simulink model "Test_Schnittstelle"  (R2018a)
settings: Solver=FixedStepAuto  StartTime=0.0  StopTime=inf  FixedStep=0.0000001  RelTol=1e-3
model workspace (MAT data in the model file):
  MCOS : class17 (value not decoded)
  MCOS : class17 (value not decoded)
  MCOS : class17 (value not decoded)
  MCOS : class17 (value not decoded)
  MCOS : class17 (value not decoded)
  MCOS : class17 (value not decoded)
  MCOS : class17 (value not decoded)
  MCOS : class17 (value not decoded)
  MCOS : class17 (value not decoded)
  MCOS : class17 (value not decoded)
  MCOS : class17 (value not decoded)
  MCOS : class17 (value not decoded)
  MCOS : class17 (value not decoded)
  MCOS : class17 (value not decoded)
  MCOS : class17 (value not decoded)
(part 2 of 2)

== matlab function Test_Schnittstelle/Schnittstelle_0/Recv_2 ==
  data: status input double size=1; clock input double size=1; lenS_1 input; lenS_2 input; lenR input; Rx_2_signal input boolean size=1; Rx_2_data input double size=[1 100]; recv_signal_2 output boolean; recv_package_2 output double size=[1 98]; Send_Buffer_1 data_store_memory; Send_Buffer_2 data_store_memory; T_send_2 data_store_memory; T_recv_2 data_store_memory; De_2 data_store_memory; De_sum_1 data_store_memory; Address data_store_memory; Recv_Buffer data_store_memory; Address_2 data_store_memory; Address_1 data_store_memory; De_sum_2 data_store_memory; Handshake_2 data_store_memory
% Name: Rx_2

% Funktionalitäten:
% Im Init-Prozess
%   1. Handshake durch zu führen
%       103...Handshake ask --> 104 in Send_Buffer_1 additieren
%       104...Handshake answer --> Handshake success
%   2. Delay-Zeit berechnen
%       105...Delay begin --> 106 in Send_Buffer_1 additieren
%       106...Delay end --> Delay_Zeit berechnen
%   3. Sum-Delay-Zeit berechnen
%       107, Receiver = meine Addresse --> Sum_Delay_Zeit berechnen
%       107, Receiver ~= meine Addresse --> Daten in Send_Buffer_2 additieren
% Im normalen Prozess
%   4. Receiver = meine Addresse --> in Recv_Buffer additieren
%   5. Receiver = 255 --> Broadcast --> in Recv_Buffer && Send_Buffer_2 additieren
%   6. Receiver ~= meine Addresse --> in Send_Buffer_2 additieren

function [recv_signal_2, recv_package_2] = Rx_2(status, clock,lenS_1, lenS_2, lenR, Rx_2_signal, Rx_2_data)

global Send_Buffer_2
global Send_Buffer_1
global T_send_2
global T_recv_2
global De_2
global De_sum_2
global Address
global Address_2
%global Address_1
global Recv_Buffer
global Handshake_2

recv_signal_2 = false;
recv_package_2 = zeros(1,98);       % one datablock = [1x7]

lenr = 1;                           % path to write data into recv_package_2

if Rx_2_signal
    a = find(Rx_2_data==102,1);
    len = a(1);
    if ~isempty(len)
        mod_ = mod(len-2,7);
        len_ = ceil((len - 2) / 7);                                 % Round toward positive infinity
    end
    
	if ((mod_ == 0) && (len_ >= 1))                             % package contains at least one datablock
        switch status
            case 1                                              % Handshake
                for i=1:len_
                    switch Rx_2_data(7*i-3)                          % Da.cmd
                        case 103                                % Handshake ask --> send answer
                            check = check_X(104, Address, Send_Buffer_1);
                            if ((Rx_2_data(7*i-5) ~= 0) && (Rx_2_data(7*i-4) == 0) && ~Handshake_2 && ~check)
                                Address_2 = Rx_2_data(7*i-5);
                                Send_Buffer_1(lenS_1:lenS_1+7) = [Address, Address_2, 104, zeros(1,4), 102];
                            end
                        case 104                                % Handshake answer --> Handshake success --> no more send
                            if ((Rx_2_data(7*i-5) ~= 0) && (Rx_2_data(7*i-4) == Address) && ~Handshake_2)
                                Address_2 = Rx_2_data(7*i-5);        % Address of the Host in the Direction_2
                                recv_package_2(lenr:lenr+6) = Rx_2_data(7*i-5:7*i+1);    % [_,_,104,_,_,_,_] = [1x7]
                                lenr = lenr + 7;
                                recv_signal_2 = true;
                            end
                    end
                end

            case 2                                              % Delay_Time_Caculation
                for j=1:len_
                    switch Rx_2_data(7*j-3)                          % Da.cmd
                        case 103                                % Handshake ask --> send answer
                            check = check_X(104, Address, Send_Buffer_1);
                            if ((Rx_2_data(7*j-5) ~= 0) && (Rx_2_data(7*j-4) == 0) && ~Handshake_2 && ~check)
                                Address_2 = Rx_2_data(7*j-5);
                                Send_Buffer_1(lenS_1:lenS_1+7) = [Address, Address_2, 104, zeros(1,4), 102];
                            end
                        case 105                                % Delay ask --> send answer
                            check = check_X(106, Address, Send_Buffer_1);
                            if (isequal(Rx_2_data(7*j-5:7*j-4),[Address_2, Address]) && Handshake_2 && ~check) % check Sender & Receiver
                                Send_Buffer_1(lenS_1:lenS_1+7) = [Address, 0, 106, zeros(1,4), 102];
                            end
                        case 106                                % Delay answer --> caculate the time --> no more send
                            if ((isequal(Rx_2_data(7*j-5:7*j-3),[Address_2, Address, 106])) && (De_2 <= 0))
                                T_recv_2 = clock;
                                De_2 = T_recv_2 - T_send_2;
                                T_send_2 = 0;
                                T_recv_2 = 0;
                            end
                    end
                end

            case 3                                              % Sum_Delay_Caculation
                for h=1:len_
                    switch Rx_2_data(7*h-3)
                        case 103                                % Handshake ask --> send answer
                            check = check_X(104, Address, Send_Buffer_1);
                            if ((Rx_2_data(7*h-5) ~= 0) && (Rx_2_data(7*h-4) == 0) && ~Handshake_2 && ~check)
                                Address_2 = Rx_2_data(7*h-5);
                                Send_Buffer_1(lenS_1:lenS_1+7) = [Address, Address_2, 104, zeros(1,4), 102];
                            end
                        case 105                                % Delay ask --> send answer
                            check = check_X(106, Address, Send_Buffer_1);
                            if (isequal(Rx_2_data(7*h-5:7*h-4),[Address_2, Address]) && Handshake_2 && ~check) % check Sender & Receiver
                                Send_Buffer_1(lenS_1:lenS_1+7) = [Address, 0, 106, zeros(1,4), 102];
                            end   
                        case 107
                            if (isequal(Rx_2_data(7*h-5:7*h-4),[Address, Address]) && (De_sum_2 <= De_2))                   % Sum_Delay --> caculate the time --> no more send
                                T_recv_2 = clock;
                                De_sum_2 = T_recv_2 - T_send_2;
                                T_send_2 = 0;
                                T_recv_2 = 0;
                            elseif ((isequal(Rx_2_data(7*h-5),Rx_2_data(7*h-4))) && (Rx_2_data(7*h-5) ~= Address))
                                check = check_Y(Rx_2_data(7*h-5:7*h), recv_package_2) && check_Y(Rx_2_data(7*h-5:7*h), Send_Buffer_2);
                                if ~check
                                    recv_package_2(lenr:lenr+6) = Rx_2_data(7*h-5:7*h+1)';
                                    lenr = lenr + 7;
                                end
                            end
                    end
                end
                Send_Buffer_2(lenS_2:lenS_2+lenr-1) = [recv_package_2(1:lenr-1),102];           % 前提：lenS更新速度比当前更新快

            case 4                                               % normal communication between all Hosts
                for k=1:len_
                    switch Rx_2_data(7*k-3)
                        case 103                                % Handshake ask --> send answer
                            check = check_X(104, Address, Send_Buffer_1);
                            if ((Rx_2_data(7*k-5) ~= 0) && (Rx_2_data(7*k-4) == 0) && ~Handshake_2 && ~check)
                                Address_2 = Rx_2_data(7*k-5);
                                Send_Buffer_1(lenS_1:lenS_1+7) = [Address, Address_2, 104, zeros(1,4), 102];
                            end
                        case 105                                % Delay ask --> send answer
                            check = check_X(106, Address, Send_Buffer_1);
                            if (isequal(Rx_2_data(7*k-5:7*k-4),[Address_2, Address]) && Handshake_2 && ~check) % check Sender & Receiver
                                Send_Buffer_1(lenS_1:lenS_1+7) = [Address, 0, 106, zeros(1,4), 102];
                            end
                        case 107
                            if ((isequal(Rx_2_data(7*k-5),Rx_2_data(7*k-4))) && (Rx_2_data(7*k-5) ~= Address))
                                check = check_Y(Rx_2_data(7*k-5:7*k), recv_package_2) && check_Y(Rx_2_data(7*k-5:7*k), Send_Buffer_2);
                                if ~check
                                    recv_package_2(lenr:lenr+6) = Rx_2_data(7*k-5:7*k+1)';
                                    lenr = lenr + 7;
                                end
                            end
                        otherwise
                            if ((Rx_2_data(7*k-5) ~= Address) && (Rx_2_data(7*k-4) == Address))   % Datablock sent to me --> store in Recv_Buffer
                                check = check_Y(Rx_2_data(7*k-5:7*k), Recv_Buffer');
                                if ~check
                                    Recv_Buffer(lenR+1,:) = Rx_2_data(7*k-5:7*k+1);
                                end
                            elseif ((Rx_2_data(7*k-5) ~=Address) && (Rx_2_data(7*k-4) == 255))    % Datablock is as a Broadcast --> store in Recv_Buffer && Send_Buffer_2
                                check = check_Y(Rx_2_data(7*k-5:7*k), Recv_Buffer');
                                if ~check
                                    Recv_Buffer(lenR+1,:) = Rx_2_data(7*k-5:7*k+1);                          % 可能存在问题，不确定lenR和本程序的更新频率
                                end
                                check = check_Y(Rx_2_data(7*k-5:7*k), recv_package_2) && check_Y(Rx_2_data(7*k-5:7*k), Send_Buffer_2);
                                if ~check
                                    recv_package_2(lenr:lenr+6) = Rx_2_data(7*k-5:7*k+1)';
                                    lenr = lenr + 7;
                                end
                            elseif ((Rx_2_data(7*k-4) ~= Address) && (Rx_2_data(7*k-4) ~= 255))   % Datablock not sent to me --> to transmmit --> store in Send_Buffer_2
                                check = check_Y(Rx_2_data(7*k-5:7*k), recv_package_2) && check_Y(Rx_2_data(7*k-5:7*k), Send_Buffer_2);
                                if ~check
                                    recv_package_2(lenr:lenr+6) = Rx_2_data(7*k-5:7*k+1)';
                                    lenr = lenr + 7;
                                end
                            end
                    end
                end
                Send_Buffer_2(lenS_2:lenS_2+lenr-1) = [recv_package_2(1:lenr-1),102];
        end
	elseif mod_ ~= 0
        fprintf("Eroor: Package length not avalueable!");
	end
end

end

function y = check_X(CMD, adr, Data)          % y: boolean; x: double, [1x100];

x = find(Data==CMD);
y = (~isempty(x));

if y
    y = y && (Data(1,x(1)-2) == adr);
end

end

function y = check_Y(data, Data)          % y: boolean; data: double, [1x6];

x = find(Data==data(3));
y = (~isempty(x));
if y
    for i=1:length(x)
        if(isequal(Data(x(i)-2:x(i)+3),data'))
            y = true;
            break
        else
            y = false;
        end
    end
end

end

== stateflow chart Test_Schnittstelle/Schnittstelle_0/Status ==
  state Init_0
    entry:	status=0;
    Handshake_1=false;
    Handshake_2=false;
    De_1 = 0;
    De_2 = 0;
    De_sum_1 = 0;
    De_sum_2 = 0;
    Filter(1,:) = zeros(1,7);
  state Error
    entry: status=-2;
  note: 未初始化全局变量
  state Init_1_Handshake
    entry: status=1;
  state Init_2_Delay_Time
    entry:	status=2;
  state Init_3_Sum_Delay_Time
    entry:	status=3;
  state Run
    entry: status=4;
  (default) -> Init_0
  Error -> Init_0 : [~Error_Signal]
  Init_0 -> Init_1_Handshake
  Init_1_Handshake -> Error [order 3] : [Error_Signal]
  Init_1_Handshake -> (junction 75) [order 1] : [recv_signal_1]
  (junction 75) -> Init_1_Handshake : [recv_data_1(1,3)==104]{Handshake_1 = true;}
  Init_1_Handshake -> (junction 77) [order 2] : [recv_signal_2]
  (junction 77) -> Init_1_Handshake : [recv_data_2(1,3)==104]{Handshake_2 = true;}
  Init_1_Handshake -> Init_2_Delay_Time [order 4] : [Handshake_1 && Handshake_2 && Address_1 > 0 && Address_2 > 0]
  Init_2_Delay_Time -> Error [order 2] : [Error_Signal]
  Init_2_Delay_Time -> Init_3_Sum_Delay_Time [order 1] : [De_1>0 && De_2>0]
  Init_3_Sum_Delay_Time -> Error [order 2] : [Error_Signal]
  Init_3_Sum_Delay_Time -> Run [order 1] : [De_sum_1 > De_1 && De_sum_2 > De_2]
  Run -> Error : [Error_Signal]
  data: status output double size=1; Error_Signal input boolean size=1; recv_signal_1 input boolean size=1; recv_data_1 input double; Handshake_1 data_store_memory size=1; Handshake_2 data_store_memory size=1; De_1 data_store_memory; De_2 data_store_memory; De_sum_1 data_store_memory; De_sum_2 data_store_memory; recv_signal_2 input boolean; recv_data_2 input double; Address_1 data_store_memory; Address_2 data_store_memory; Filter data_store_memory

== matlab function Test_Schnittstelle/MATLAB Function ==
  data: u input; y output; u_old input
function y  = fcn(u,u_old)

if u_old
    y = false;
else
    y = u;
end
end

== matlab function Test_Schnittstelle/Schnittstelle_0/Send_to_Host ==
  data: signal output boolean size=1; package output double; Recv_Buffer data_store_memory; Filter data_store_memory; lenR input; lenF input; signal_old input
% Name: Send_to_Host
% Funktionalitäten:
% 1. Erste Zeile der Nachricht von Recv_Buffer in Filter prüfen
% 2. nicht wiederholte Nachricht an Host senden
% 3. wiederholte Nachricht in Filter löschen
% 4. gesendete Nachricht in Filter kopieren
% 5. folgende Nachrichten eine Zeile nach oben verschoben


function [signal, package] = send_to_Host(lenR, lenF, signal_old)

global Recv_Buffer          % Package-List, which will be sent to the Host
global Filter               % Package-List, which has been sent to the Host

package = zeros(1,7);
check = 0;

if signal_old               % signal can only last for one periode
    signal = false;
    package = zeros(1,7);

else                        % signal inactiv --> now we can send new data to host.
    if (lenR >= 1)
        if lenF >= 1        % check in Filter
            for i=1:lenF        % check if the same message sent before
                if isequal(Recv_Buffer(1,:),Filter(i,:))
                    check = i;
                    break
                else
                    check = 0;
                end
            end
        end
        
        if check ~= 0       % same message in Filter found --> delete the message in Recv_Buffer and Filter
            signal = false;
            package = zeros(1,7);
            Filter(check:lenF-1,:) = Filter(check+1:lenF,:);
            Filter(lenF,:) = zeros(1,7);
            Recv_Buffer(1:lenR-1,:) = Recv_Buffer(2:lenR,:);
            Recv_Buffer(lenR,:) = zeros(1,7);
        else                % same message in Filter not found --> send to Host --> copy the message in Filter delete it in Recv_Buffer
            package = Recv_Buffer(1,:);
            signal = true;
            Filter(lenF+1,:) = Recv_Buffer(1,:);    % copy
            Recv_Buffer(1:lenR-1,:) = Recv_Buffer(2:lenR,:);    % delete
            Recv_Buffer(lenR,:) = zeros(1,7);
        end
    else
        signal = false;
        package = zeros(1,7);
    end
end


end

== matlab function Test_Schnittstelle/Schnittstelle_0/Global_Var_Length ==
  data: len_Send_Buffer_1 output double size=1; len_Send_Buffer_2 output double size=1; len_Recv_Buffer output double size=1; len_Filter output double size=1; Send_Buffer_1 data_store_memory; Send_Buffer_2 data_store_memory; Recv_Buffer data_store_memory; Filter data_store_memory
% genutzte Länge der globale Variablen berechnen

function [len_Send_Buffer_1, len_Send_Buffer_2, len_Recv_Buffer, len_Filter] = Length
global Send_Buffer_1
global Send_Buffer_2
global Recv_Buffer
global Filter

a1 = find(Send_Buffer_1==102,1);
len_Send_Buffer_1 = a1(1);
a2 = find(Send_Buffer_2==102,1);
len_Send_Buffer_2 = a2(1);

len_Recv_Buffer = min(find(Recv_Buffer==0,150))-1;
len_Filter = min(find(Filter(2:20)==0,150));

end

== matlab function Test_Schnittstelle/MATLAB Function1 ==
  data: u input; y output; u_old input
function y  = fcn(u,u_old)

if u_old
    y = false;
else
    y = u;
end
end
